simulink model "Assignment_2_PacemakerProjRA"  (R2022b)
settings: Solver=FixedStepAuto  StartTime=0.0  StopTime=30  FixedStep=1e-3  RelTol=1e-3  EnableMultiTasking=on
undefined symbols (not defined in the file): A0, A1, D0, D1, D10, D11, D12, D13, D2, D3, D4, D5, D6, D7, D8, D9, PTA0, PTA1, PTA2, PTB2, PTB23, PTB3, PTB9, PTC16, PTC17, PTC2, PTC3, PTC4, PTD0, PTD1, PTD2, PTD3
libraries: frdmk64flib x22, etargetslib x8, simulink x4
settings Model: ExtModeTrigDuration=5  Creator=varun  LastModifiedBy=lupas
settings SolverCC: AutoInsertRateTranBlk=on
settings OptimizationCC: EnhancedBackFolding=on  PassReuseOutputArgsAs=Individual arguments  ZeroExternalMemoryAtStartup=off  ZeroInternalMemoryAtStartup=off  MaxStackSize=64  OptimizeBlockOrder=speed  DifferentSizesBufferReuse=on  OptimizationCustomize=off  EfficientTunableParamExpr=on
settings DebuggingCC: ParameterTunabilityLossMsg=error
settings HardwareCC: ProdBitPerPointer=32  ProdBitPerSizeT=32  ProdBitPerPtrDiffT=32  ProdLargestAtomicInteger=Long  ProdLargestAtomicFloat=Double  ProdWordSize=32  ProdHWDeviceType=ARM Compatible->ARM Cortex
settings SFSimCC: MATLABDynamicMemAlloc=off
settings RTWCC: Description=Embedded Coder  SystemTargetFile=ert.tlc  HardwareBoard=NXP FRDM-K64F  TLCOptions="-aInlineSetEventsForThisBaseRateFcn=TLC_FALSE -aSuppressMultiTaskScheduler=TLC_FALSE  -aRateBasedStepFcn=0"  TemplateMakefile=ert_default_tmf  Toolchain=GNU Tools for ARM Embedded Processors
settings CodeAppCC: ForceParamTrailComments=on  IgnoreCustomStorageClasses=off  OperatorAnnotations=on  SimulinkDataObjDesc=on  SFDataObjDesc=on  InsertBlockDesc=on
settings ERTTargetCC: ExtModeTransport=4  ExtModeMexFile=sendToCommService

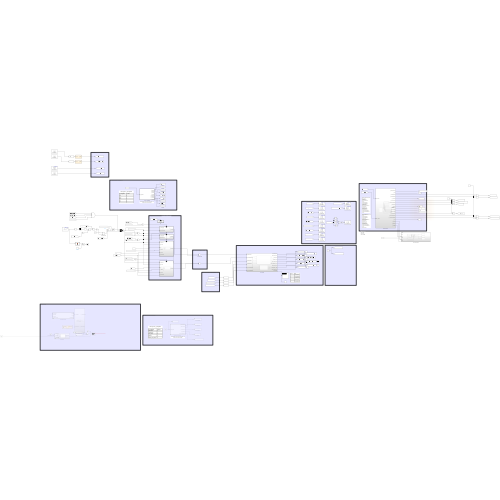
[thumbnail: Simulink's stored preview of the top-level diagram]
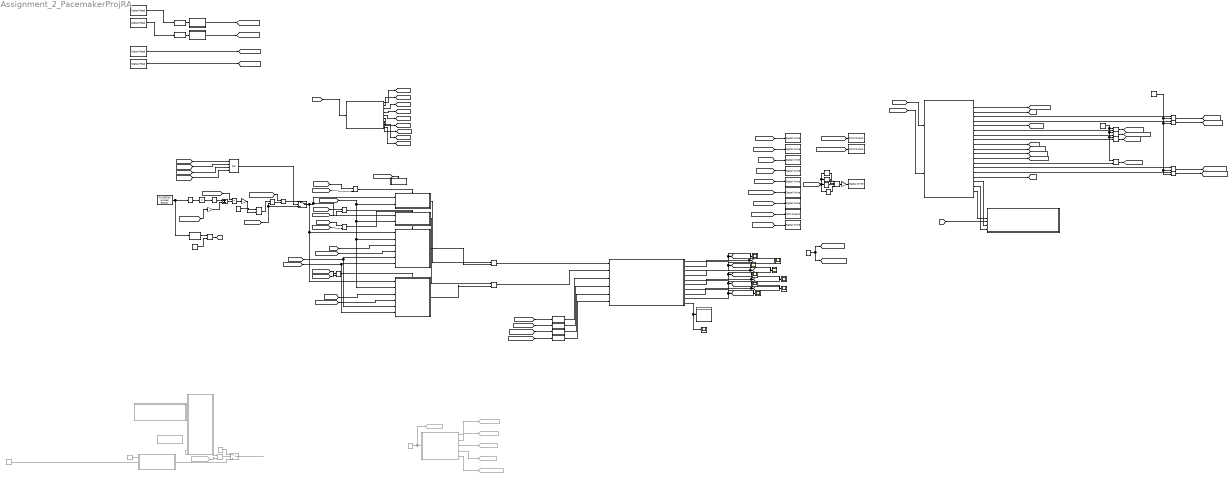
== system Assignment_2_PacemakerProjRA ==
  note: p_currentState:
      | 0x20 = Write
      | 0x16 = Echo
      | 0x22 = EGRAM
  note: Pace Making Code
  note: 'Input Variables
  note: Unused functions
  note: REF_PWM setter
  note: Output Pins
  note: Pacing System Programmable Variables
  note: Output
      | State
      |
      | 1
      | y_atriumPaced
      |
      | 2
      | y_ventriclePaced
      |
      | 3
      | y_initialDischarge
      |
      | 4
      | y_c22Charged
      |
      | 5
      | y_pulseReceived
  note: Atrial and Ventricular Pacing Signals
  note: Decoding and defining Pacing States
  note: Decoding and defining Pacing Modes
  note: Simple MATLAB code to convert input integer into a boolean set of output variables
  note: Taken from: Page 16 - Section 3.5
  note: Units/Type for y_pacingMode
      |
      | p_pacingMode
      | Int Value
      |
      | OFF
      | 0
      |
      | AOO
      | 1
      |
      | VOO
      | 2
      |
      | AAI
      | 3
      |
      | VVI
      | 4
  note: Pacing Modes
  note: Units/Type for y_pacingState
      |
      | p_pacingMode
      | Int Value
      |
      | PERMANENT
      | 0
      |
      | TEMPORARY
      | 1
      |
      | PACE_NOW
      | 2
      |
      | MAGNET
      | 3
      |
      | POWER_ON_RESET
      | 4
  note: Simple MATLAB code to convert input integer into a boolean set of output variables
  note: Number of Bytes for Input: 24
      | sync: 1 (16)
      | p_currentState: 1
      | p_mode: 1
      | p_activityThreshold: 1
      | p_arp: 2
      | p_atrialAmplitude: 2
      | p_atrialPulseWidth: 2
      | p_hysteresis: 1
      | p_hysteresisLimit: 1
      | p_maximumSensorRate: 1
      | p_lowrateLimit: 1
      | p_reactionTime: 1
      | p_recoveryTime: 1
      | p_responseFactor: 1
      | p_upperrateLimit: 1
      | p_ventricularAmplitude: 2
      | p_ventricularPulseWidth: 2
      | p_vrp: 2
  note: Input and Output for UART
  note: Number of Bytes for Output: 26
      | p_activityThreshold: 1
      | p_arp: 2
      | p_atrialAmplitude: 2
      | p_atrialPulseWidth: 2
      | p_hysteresis: 1
      | p_hysteresisLimit: 1
      | p_maximumSensorRate: 1
      | p_lowrateLimit: 1
      | p_reactionTime: 1
      | p_recoveryTime: 1
      | p_responseFactor: 1
      | p_upperrateLimit: 1
      | p_ventricularAmplitude: 2
      | p_ventricularPulseWidth: 2
      | p_vrp: 2
      | The two signals
  AAI : Subsystem
  AOO : Subsystem
  Chart : Stateflow chart  TreatAsAtomicUnit=on
  Chart1 : Stateflow chart  TreatAsAtomicUnit=on
  Compare To Constant : simulink/Logic and Bit Operations/Compare To Constant  relop===  const=3  OutDataTypeStr=boolean
  Compare To Constant1 : simulink/Logic and Bit Operations/Compare To Constant  relop===  const=4  OutDataTypeStr=boolean
  Compare To Constant2 : simulink/Logic and Bit Operations/Compare To Constant  relop===  const=7  OutDataTypeStr=boolean
  Compare To Constant3 : simulink/Logic and Bit Operations/Compare To Constant  relop===  const=8  OutDataTypeStr=boolean
  Constant : Constant  Value=0.8
  Constant1 : Constant  Value=70
  Constant19 : Constant  Commented=on  Value=0.4  OutDataTypeStr=single
  Constant20 : Constant  Commented=on  Value=.5
  Constant4 : Constant  Value=1000
  Constant5 : Constant  Value=60000
  Constant6 : Constant  Value=60000
  Cool Colour Effects : Subsystem
  Data Processing : Subsystem
  Data Type Conversion : DataTypeConversion  OutDataTypeStr=uint16  SaturateOnIntegerOverflow=off  RndMeth=Floor
  Data Type Conversion1 : DataTypeConversion  OutDataTypeStr=uint16  SaturateOnIntegerOverflow=off  RndMeth=Floor
  Data Type Conversion{2..5} (4 alike) : DataTypeConversion  OutDataTypeStr=double  SaturateOnIntegerOverflow=off  RndMeth=Floor
  Decode p_pacingMode : MATLAB Function  TreatAsAtomicUnit=on
  Decode p_pacingState : MATLAB Function  Commented=on  TreatAsAtomicUnit=on
  Digital Read : frdmk64flib/Digital Read  Whichpin=PTC16 (D0)  SampleTime=-1
  Digital Read1 : frdmk64flib/Digital Read  Whichpin=PTC17 (D1)  SampleTime=-1
  Digital Read2 : frdmk64flib/Digital Read  Whichpin=PTB2 (A0)  SampleTime=-1
  Digital Read3 : frdmk64flib/Digital Read  Whichpin=PTB3 (A1)  SampleTime=-1
  Digital Write : frdmk64flib/Digital Write  Whichpin=PTD2 (D11)
  Digital Write1 : frdmk64flib/Digital Write  Whichpin=PTD3 (D12)
  Digital Write2 : frdmk64flib/Digital Write  Whichpin=PTB23 (D4)
  Digital Write3 : frdmk64flib/Digital Write  Whichpin=PTC3 (D7)
  Digital Write4 : frdmk64flib/Digital Write  Whichpin=PTA0 (D8)
  Digital Write5 : frdmk64flib/Digital Write  Whichpin=PTB9 (D2)
  Digital Write6 : frdmk64flib/Digital Write  Whichpin=PTD0 (D10)
  Digital Write8 : frdmk64flib/Digital Write  Whichpin=PTC4 (D9)
  Digital Write9 : frdmk64flib/Digital Write  Whichpin=PTD1 (D13)
  Display : Display
  Divide{,1..7} (8 alike) : Product  Inputs=*/
  FXOS8700 6-Axes Sensor1 : frdmk64flib/FXOS8700 6-Axes Sensor  Activesensor=Accelerometer only  ODR=800Hz  HybridODR=400Hz  Accelfullrange=-4g to +4g  SampleTime=-1
  Float Variable6 : Subsystem  Commented=on
  From52 : From  Commented=on  GotoTag=s_paceNowState
  From53 : From  Commented=on  GotoTag=s_powerOnResetState
  Gain : Gain  Gain=0.5
  Gain1 : Gain  Gain=4
  Goto28 : Goto  Commented=on  GotoTag=p_currentState
  GreaterThan : RelationalOperator  OutDataTypeStr=boolean  RndMeth=Simplest  InputSameDT=off
  Lowrate Upperrate Limit Checker1 : Subsystem  Commented=on
  MATLAB Function1 : MATLAB Function  TreatAsAtomicUnit=on
  Max1 : MinMax  Inputs=2
  Min1 : MinMax  Function=max  Inputs=2
  Minus1 : Sum  Inputs=+-
  Multiply : Gain  Gain=3.3  OutDataTypeStr=double
  OFF : Subsystem
  OR : Logic  Operator=OR  Inputs=4  IconShape=distinctive  AllPortsSameDT=off  OutDataTypeStr=boolean
  OR{1..4} (4 alike) : Logic  Operator=OR  IconShape=distinctive  AllPortsSameDT=off  OutDataTypeStr=boolean
  OR5 : Logic  Operator=OR  Inputs=4  IconShape=distinctive  AllPortsSameDT=off  OutDataTypeStr=boolean
  OR8 : Logic  Commented=on  Operator=OR  IconShape=distinctive  AllPortsSameDT=off  OutDataTypeStr=boolean
  PWM Output : frdmk64flib/PWM Output  Whichpin=PTA1 (D3)  InitialFrequency=2000  InitialDutyCycle=50
  PWM Output1 : frdmk64flib/PWM Output  Whichpin=PTA2 (D5)  InitialFrequency=2000  InitialDutyCycle=50
  PWM Output2 : frdmk64flib/PWM Output  Whichpin=PTC2 (D6)  InitialFrequency=2000  InitialDutyCycle=50
  Pacing System : Subsystem
  Product : Product
  Scope{,2..10} (10 alike) : Scope
  Sqrt : Sqrt
  Square : Math  Operator=square
  Sum of Elements : Sum  Inputs=+
  Switch : Switch  Criteria=u2 > Threshold  SaturateOnIntegerOverflow=off  InputSameDT=off
  Switch7 : Switch  Commented=on  Criteria=u2 > Threshold  OutDataTypeStr=single  SaturateOnIntegerOverflow=off  InputSameDT=off
  VOO : Subsystem
  VVI : Subsystem
  Write Mode : Stateflow chart  Commented=on  TreatAsAtomicUnit=on
  checkRangeFunction7 : MATLAB Function  Commented=on  TreatAsAtomicUnit=on
  p_lowrateInterval1 : Product  Inputs=*/
  p_pacingState : Constant  Commented=on  Value=0  OutDataTypeStr=uint8
  p_ventricularPulseWidth1 : Constant  Commented=on  Value=0.4  OutDataTypeStr=single
  s_atrialPaceStart : Logic  Operator=OR  IconShape=distinctive  AllPortsSameDT=off  OutDataTypeStr=boolean
  s_magnetState : Goto  Commented=on  GotoTag=s_magnetState
  s_paceNowState : Goto  Commented=on  GotoTag=s_paceNowState
  s_permanentState : Goto  Commented=on  GotoTag=s_permanentState
  s_powerOnResetState : Goto  Commented=on  GotoTag=s_powerOnResetState
  s_temporaryState : Goto  Commented=on  GotoTag=s_temporaryState
  s_ventricularPaceStart : Logic  Operator=OR  IconShape=distinctive  AllPortsSameDT=off  OutDataTypeStr=boolean
  wires:
  [s_offState] -> OFF/Enable
  Decode p_pacingMode/1(s_offState) -> [s_offState]
  Decode p_pacingMode/2(s_AOOState) -> [s_AOOState]
  Decode p_pacingMode/4(s_AAIState) -> [s_AAIState]
  Decode p_pacingMode/5(s_VVIState) -> [s_VVIState]
  Decode p_pacingMode/3(s_VOOState) -> [s_VOOState]
  p_pacingState/1 -> Goto28/1, Decode p_pacingState/1(p_pacingState)
  Decode p_pacingState/1(s_permanentState) -> s_permanentState/1
  Decode p_pacingState/2(s_temporaryState) -> s_temporaryState/1
  Decode p_pacingState/3(s_paceNowState) -> s_paceNowState/1
  Decode p_pacingState/4(s_magnetState) -> s_magnetState/1
  Decode p_pacingState/5(S_powerOnResetState) -> s_powerOnResetState/1
  OR3/1 -> AAI/Enable
  OR4/1 -> VVI/Enable
  s_atrialPaceStart/1 -> Pacing System/1(s_atrialPaceStart)
  [p_atrialAmplitude] -> Data Type Conversion5/1
  [p_atrialPulseWidth] -> Data Type Conversion4/1
  [p_ventricularAmplitude] -> Data Type Conversion3/1
  [p_ventricularPulseWidth] -> Data Type Conversion2/1
  s_ventricularPaceStart/1 -> Pacing System/2(s_ventricularPaceStart)
  Pacing System/1(ATR_GND_CTRL) -> [ATR_GND_CTRL], Scope2/1
  Pacing System/3(Z_ATR_CTRL) -> [Z_ATR_CTRL], Scope4/1
  Pacing System/2(VENT_GND_CTRL) -> [VENT_GND_CTRL], Scope3/1
  Pacing System/4(Z_VENT_CTRL) -> Scope5/1, [Z_VENT_CTRL]
  Pacing System/6(PACE_CHARGE_CTRL) -> Scope7/1, [PACE_CHARGE_CTRL]
  Pacing System/5(ATR_PACE_CTRL) -> [ATR_PACE_CTRL], Scope6/1
  Pacing System/7(PACE_GND_CTRL) -> Scope8/1, [PACE_GND_CTRL]
  Pacing System/9(VENT_PACE_CTRL) -> [VENT_PACE_CTRL], Scope10/1
  Pacing System/8(PACING_REF_PWM) -> Scope9/1, [PACING_REF_PWM]
  Pacing System/10(Visual Output) -> Scope/1, Display/1
  [VENT_PACE_CTRL] -> Digital Write8/1
  [PACING_REF_PWM] -> PWM Output1/1
  [PACE_GND_CTRL] -> Digital Write6/1
  [PACE_CHARGE_CTRL] -> Digital Write5/1
  [ATR_PACE_CTRL] -> Digital Write4/1
  [Z_VENT_CTRL] -> Digital Write3/1
  [Z_ATR_CTRL] -> Digital Write2/1
  [VENT_GND_CTRL] -> Digital Write1/1
  [ATR_GND_CTRL] -> Digital Write/1
  OR1/1 -> AOO/Enable
  OR2/1 -> VOO/Enable
  AOO/1(s_paceStart) -> s_atrialPaceStart/1
  VOO/1(s_paceStart) -> s_ventricularPaceStart/1
  Digital Read/1 -> [ATR_CMP_DETECT]
  Digital Read1/1 -> [VENT_CMP_DETECT]
  [ATR_CMP_REF_PWM] -> PWM Output2/1
  [VENT_CMP_REF_PWM] -> PWM Output/1
  Constant1/1 -> [ATR_CMP_REF_PWM], [VENT_CMP_REF_PWM]
  OR/1 -> Multiply/1
  Compare To Constant/1 -> OR/1
  Compare To Constant1/1 -> OR/2
  Multiply/1 -> Digital Write9/1
  [p_mode] -> Compare To Constant3/1, Compare To Constant2/1, Compare To Constant1/1, Compare To Constant/1
  AAI/1(s_paceStart) -> s_atrialPaceStart/2
  VVI/1(s_paceStart) -> s_ventricularPaceStart/2
  [p_upperrateLimit] -> AOO/2(p_uppperrateInterval), VOO/2(p_uppperrateInterval), VVI/2(p_upperLimit), AAI/2(p_upperLimit)
  [ATR_CMP_DETECT] -> AAI/4(m_atrSense)
  [p_arp] -> AAI/3(p_arp)
  [p_vrp] -> VVI/3(p_vrp)
  [VENT_CMP_DETECT] -> VVI/4(m_ventSense)
  Data Type Conversion2/1 -> Pacing System/6(p_ventricularPulseWidth)
  Data Type Conversion3/1 -> Pacing System/5(p_ventricularAmplitude)
  Data Type Conversion4/1 -> Pacing System/4(p_atrialPulseWidth)
  Data Type Conversion5/1 -> Pacing System/3(p_atrialAmplitude)
  Constant20/1 -> Switch7/1
  Float Variable6/1(p_outputValue) -> Switch7/3
  From53/1 -> OR8/1
  OR8/1 -> Switch7/2
  From52/1 -> OR8/2
  Constant19/1 -> Float Variable6/2(m_newValue)
  p_ventricularPulseWidth1/1 -> Float Variable6/1(k_defaultValue)
  Switch7/1 -> ?
  [p_mode] -> Decode p_pacingMode/1(p_pacingMode)
  Divide2/1 -> [p_upperrateLimit]
  Divide1/1 -> [p_maximumSensorRate]
  Divide/1 -> [p_lowrateLimit]
  Constant5/1 -> Divide7/1, Divide2/1, Divide/1, Divide1/1
  Data Processing/1(p_activityThreshold1) -> [p_activityThreshold]
  Data Processing/2(p_arp1) -> [p_arp]
  Data Processing/3(p_atrialAmplitude1) -> Divide3/1
  Data Processing/4(p_atrialPulseWidth1) -> Divide4/1
  Data Processing/5(p_hysteresis1) -> [p_hysteresis]
  Data Processing/7(p_maximumSensorRate1) -> Divide1/2
  Data Processing/8(p_lowrateLimit1) -> Divide/2
  Data Processing/10(p_reactionTime1) -> [p_reactionTime]
  Data Processing/11(p_recoveryTime1) -> [p_recoveryTime]
  Data Processing/12(p_responseFactor1) -> [p_responseFactor]
  Data Processing/13(p_upperrateLimit1) -> Divide2/2
  Data Processing/14(p_ventricularAmplitude1) -> Divide5/1
  Data Processing/15(p_ventricularPulseWidth1) -> Divide6/1
  Data Processing/16(p_vrp1) -> [p_vrp]
  Data Processing/18(p_uartGreen) -> Cool Colour Effects/6(Green)
  Data Processing/19(p_uartBlue) -> Cool Colour Effects/3(Blue)
  Data Processing/17(p_uartRed) -> Cool Colour Effects/5(Red)
  Data Processing/9(p_mode1) -> [p_mode]
  Divide3/1 -> [p_atrialAmplitude]
  Divide4/1 -> [p_atrialPulseWidth]
  Constant4/1 -> Divide6/2, Divide5/2, Divide4/2, Divide3/2
  Divide6/1 -> [p_ventricularPulseWidth]
  Divide5/1 -> [p_ventricularAmplitude]
  Data Processing/6(p_hysteresisLimit1) -> Divide7/2
  [p_hysteresis] -> VVI/5(p_hysteresis), AAI/5(p_hysteresis)
  [p_hysteresisLimit] -> VVI/6(p_hysteresisLimit), AAI/6(p_hysteresisLimit)
  Digital Read3/1 -> Data Type Conversion1/1
  Digital Read2/1 -> Data Type Conversion/1
  [ATR_SIGNAL] -> Data Processing/1(ATR_SIGNAL)
  [VENT_SIGNAL] -> Data Processing/2(VENT_SIGNAL)
  Divide7/1 -> [p_hysteresisLimit]
  Data Type Conversion/1 -> Chart/1(m_input)
  Data Type Conversion1/1 -> Chart1/1(m_input)
  Chart/1(p_output) -> [ATR_SIGNAL]
  Chart1/1(p_output) -> [VENT_SIGNAL]
  Decode p_pacingMode/6(s_AOORState) -> [s_AOORState]
  Decode p_pacingMode/7(s_VOORState) -> [s_VOORState]
  Decode p_pacingMode/8(s_AAIRState) -> [s_AAIRState]
  Decode p_pacingMode/9(s_VVIRState) -> [s_VVIRState]
  [s_AOOState] -> OR1/2
  [s_AOORState] -> OR1/1
  [s_VOOState] -> OR2/2
  [s_VOORState] -> OR2/1
  [s_AAIState] -> OR3/2
  [s_AAIRState] -> OR3/1
  [s_VVIState] -> OR4/1
  [s_VVIRState] -> OR4/2
  [s_VVIRState] -> OR5/4
  [s_AAIRState] -> OR5/3
  [s_VOORState] -> OR5/2
  [s_AOORState] -> OR5/1
  Compare To Constant2/1 -> OR/3
  Compare To Constant3/1 -> OR/4
  FXOS8700 6-Axes Sensor1/1 -> MATLAB Function1/1(u), Square/1
  MATLAB Function1/1(y) -> GreaterThan/1
  GreaterThan/1 -> [SUS]
  Constant/1 -> GreaterThan/2
  [SUS] -> Cool Colour Effects/4(Yellow)
  OR5/1 -> Switch/2
  Minus1/1 -> Product/2
  [p_maximumSensorRate] -> Min1/1
  Constant6/1 -> p_lowrateInterval1/1
  Product/1 -> Gain1/1
  Sqrt/1 -> Minus1/1
  Square/1 -> Sum of Elements/1
  Max1/1 -> Min1/2
  [p_lowrateLimit] -> Switch/3, Max1/2
  Sum of Elements/1 -> Sqrt/1
  [p_responseFactor] -> Product/1
  Gain/1 -> Minus1/2
  [p_activityThreshold] -> Gain/1
  Gain1/1 -> p_lowrateInterval1/2
  p_lowrateInterval1/1 -> Max1/1
  Min1/1 -> Switch/1
  Switch/1 -> VVI/1(p_lowrateLimit), AAI/1(p_lowrateLimit), VOO/1(p_lowrateInterval), AOO/1(p_lowrateInterval)

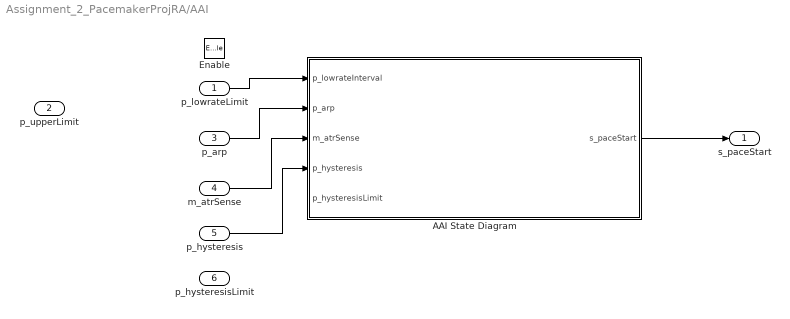
== system Assignment_2_PacemakerProjRA/AAI ==
  p_lowrateLimit : Inport
  p_upperLimit : Inport  Port=2
  p_arp : Inport  Port=3
  m_atrSense : Inport  Port=4
  p_hysteresis : Inport  Port=5
  p_hysteresisLimit : Inport  Port=6
  Enable : EnablePort
  AAI State Diagram : Stateflow chart  TreatAsAtomicUnit=on
  s_paceStart : Outport
  wires:
  p_lowrateLimit/1 -> AAI State Diagram/1(p_lowrateInterval)
  AAI State Diagram/1(s_paceStart) -> s_paceStart/1
  m_atrSense/1 -> AAI State Diagram/3(m_atrSense)
  p_arp/1 -> AAI State Diagram/2(p_arp)
  p_hysteresis/1 -> AAI State Diagram/4(p_hysteresis)

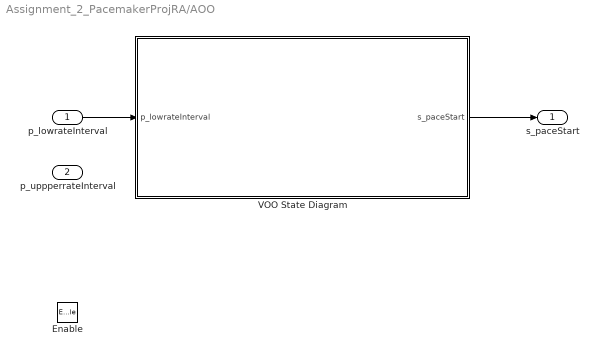
== system Assignment_2_PacemakerProjRA/AOO ==
  p_lowrateInterval : Inport
  p_uppperrateInterval : Inport  Port=2
  Enable : EnablePort
  VOO State Diagram : Stateflow chart  TreatAsAtomicUnit=on
  s_paceStart : Outport
  wires:
  p_lowrateInterval/1 -> VOO State Diagram/1(p_lowrateInterval)
  VOO State Diagram/1(s_paceStart) -> s_paceStart/1

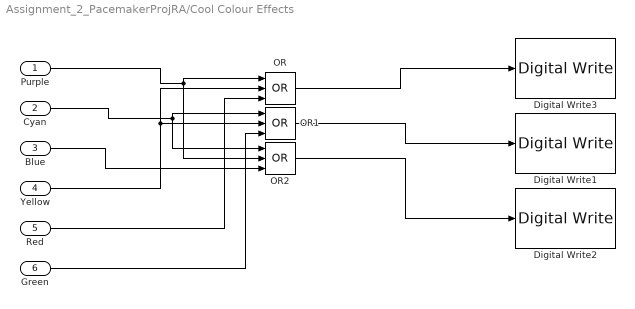
== system Assignment_2_PacemakerProjRA/Cool Colour Effects ==
  Purple : Inport
  Cyan : Inport  Port=2
  Blue : Inport  Port=3
  Yellow : Inport  Port=4
  Red : Inport  Port=5
  Green : Inport  Port=6
  Digital Write1 : frdmk64flib/Digital Write  Whichpin=GREEN_LED
  Digital Write2 : frdmk64flib/Digital Write  Whichpin=BLUE_LED
  Digital Write3 : frdmk64flib/Digital Write  Whichpin=RED_LED
  OR : Logic  Operator=OR  Inputs=3  IconShape=distinctive  AllPortsSameDT=off  OutDataTypeStr=boolean
  OR1 : Logic  Operator=OR  Inputs=3  IconShape=distinctive  AllPortsSameDT=off  OutDataTypeStr=boolean
  OR2 : Logic  Operator=OR  Inputs=3  IconShape=distinctive  AllPortsSameDT=off  OutDataTypeStr=boolean
  wires:
  Blue/1 -> OR2/3
  Cyan/1 -> OR2/1, OR1/1
  Purple/1 -> OR2/2, OR/1
  Yellow/1 -> OR1/2, OR/2
  Red/1 -> OR/3
  Green/1 -> OR1/3
  OR/1 -> Digital Write3/1
  OR2/1 -> Digital Write2/1
  OR1/1 -> Digital Write1/1

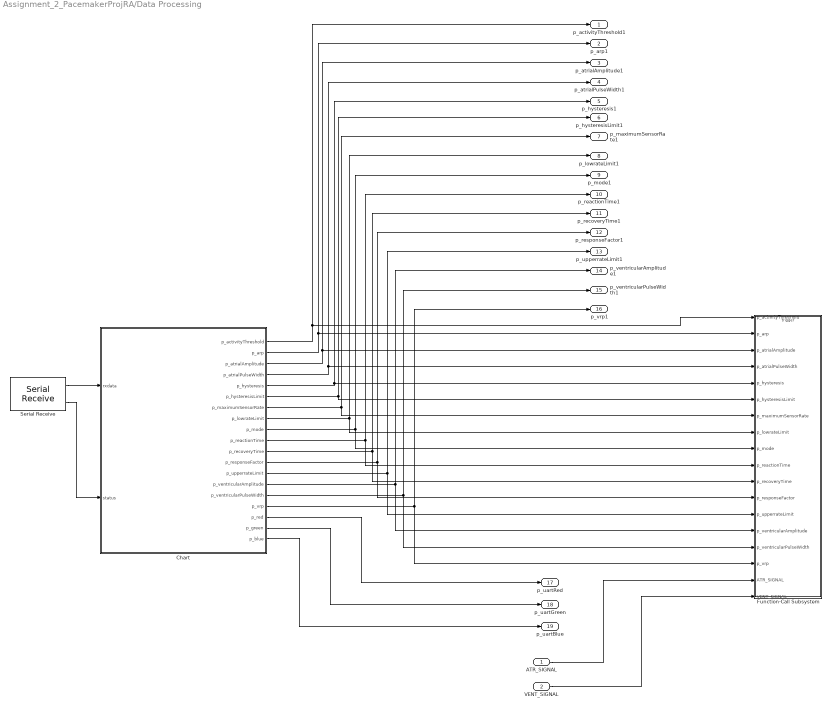
== system Assignment_2_PacemakerProjRA/Data Processing ==
  ATR_SIGNAL : Inport  OutDataTypeStr=uint16
  VENT_SIGNAL : Inport  Port=2  OutDataTypeStr=uint16
  Chart : Stateflow chart  TreatAsAtomicUnit=on
  Function-Call Subsystem : Subsystem  TreatAsAtomicUnit=on
  Serial Receive : frdmk64flib/Serial Receive  SCIModule=0  Baudrate=uint32(9600)  Parity=None  StopBits=1  HardwareFlowControl=None  ByteOrder=LittleEndian  DataType=uint8  DataLength=24  BlockingMode=off  OutputStatus=on  SampleTime=0.1
  p_activityThreshold1 : Outport
  p_arp1 : Outport  Port=2
  p_atrialAmplitude1 : Outport  Port=3
  p_atrialPulseWidth1 : Outport  Port=4
  p_hysteresis1 : Outport  Port=5
  p_hysteresisLimit1 : Outport  Port=6
  p_maximumSensorRate1 : Outport  Port=7
  p_lowrateLimit1 : Outport  Port=8
  p_mode1 : Outport  Port=9
  p_reactionTime1 : Outport  Port=10
  p_recoveryTime1 : Outport  Port=11
  p_responseFactor1 : Outport  Port=12
  p_upperrateLimit1 : Outport  Port=13
  p_ventricularAmplitude1 : Outport  Port=14
  p_ventricularPulseWidth1 : Outport  Port=15
  p_vrp1 : Outport  Port=16
  p_uartRed : Outport  Port=17
  p_uartGreen : Outport  Port=18
  p_uartBlue : Outport  Port=19
  wires:
  Serial Receive/1 -> Chart/1(rxdata)
  Serial Receive/2 -> Chart/2(status)
  Chart/17(p_red) -> p_uartRed/1
  Chart/18(p_green) -> p_uartGreen/1
  Chart/19(p_blue) -> p_uartBlue/1
  Chart/11(p_recoveryTime) -> p_recoveryTime1/1, Function-Call Subsystem/11(p_recoveryTime)
  Chart/14(p_ventricularAmplitude) -> p_ventricularAmplitude1/1, Function-Call Subsystem/14(p_ventricularAmplitude)
  Chart/3(p_atrialAmplitude) -> p_atrialAmplitude1/1, Function-Call Subsystem/3(p_atrialAmplitude)
  Chart/2(p_arp) -> p_arp1/1, Function-Call Subsystem/2(p_arp)
  Chart/7(p_maximumSensorRate) -> p_maximumSensorRate1/1, Function-Call Subsystem/7(p_maximumSensorRate)
  Chart/15(p_ventricularPulseWidth) -> p_ventricularPulseWidth1/1, Function-Call Subsystem/15(p_ventricularPulseWidth)
  Chart/9(p_mode) -> p_mode1/1, Function-Call Subsystem/9(p_mode)
  Chart/8(p_lowrateLimit) -> p_lowrateLimit1/1, Function-Call Subsystem/8(p_lowrateLimit)
  Chart/4(p_atrialPulseWidth) -> p_atrialPulseWidth1/1, Function-Call Subsystem/4(p_atrialPulseWidth)
  Chart/13(p_upperrateLimit) -> p_upperrateLimit1/1, Function-Call Subsystem/13(p_upperrateLimit)
  Chart/12(p_responseFactor) -> p_responseFactor1/1, Function-Call Subsystem/12(p_responseFactor)
  Chart/1(p_activityThreshold) -> p_activityThreshold1/1, Function-Call Subsystem/1(p_activityThreshold)
  Chart/5(p_hysteresis) -> p_hysteresis1/1, Function-Call Subsystem/5(p_hysteresis)
  Chart/16(p_vrp) -> p_vrp1/1, Function-Call Subsystem/16(p_vrp)
  Chart/10(p_reactionTime) -> p_reactionTime1/1, Function-Call Subsystem/10(p_reactionTime)
  Chart/6(p_hysteresisLimit) -> p_hysteresisLimit1/1, Function-Call Subsystem/6(p_hysteresisLimit)
  ATR_SIGNAL/1 -> Function-Call Subsystem/17(ATR_SIGNAL)
  VENT_SIGNAL/1 -> Function-Call Subsystem/18(VENT_SIGNAL)

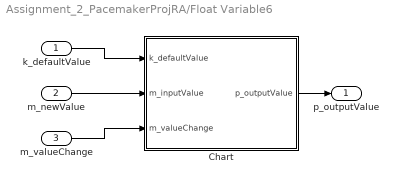
== system Assignment_2_PacemakerProjRA/Float Variable6 ==
  k_defaultValue : Inport
  m_newValue : Inport  Port=2
  m_valueChange : Inport  Port=3
  Chart : Stateflow chart  TreatAsAtomicUnit=on
  p_outputValue : Outport
  wires:
  Chart/1(p_outputValue) -> p_outputValue/1
  m_newValue/1 -> Chart/2(m_inputValue)
  k_defaultValue/1 -> Chart/1(k_defaultValue)
  m_valueChange/1 -> Chart/3(m_valueChange)

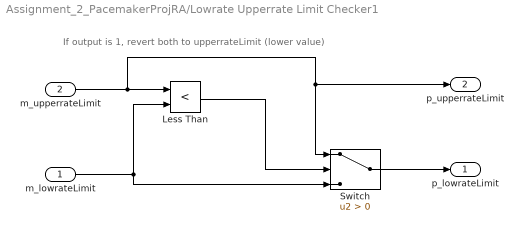
== system Assignment_2_PacemakerProjRA/Lowrate Upperrate Limit Checker1 ==
  note: If output is 1, revert both to upperrateLimit (lower value)
  m_lowrateLimit : Inport
  m_upperrateLimit : Inport  Port=2
  Less Than : RelationalOperator  Operator=<  OutDataTypeStr=boolean  RndMeth=Simplest  InputSameDT=off
  Switch : Switch  Criteria=u2 > Threshold  SaturateOnIntegerOverflow=off  InputSameDT=off
  p_lowrateLimit : Outport  OutDataTypeStr=single
  p_upperrateLimit : Outport  Port=2  OutDataTypeStr=single
  wires:
  m_upperrateLimit/1 -> Switch/1, p_upperrateLimit/1, Less Than/1
  m_lowrateLimit/1 -> Switch/3, Less Than/2
  Switch/1 -> p_lowrateLimit/1
  Less Than/1 -> Switch/2

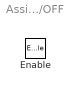
== system Assignment_2_PacemakerProjRA/OFF ==
  Enable : EnablePort

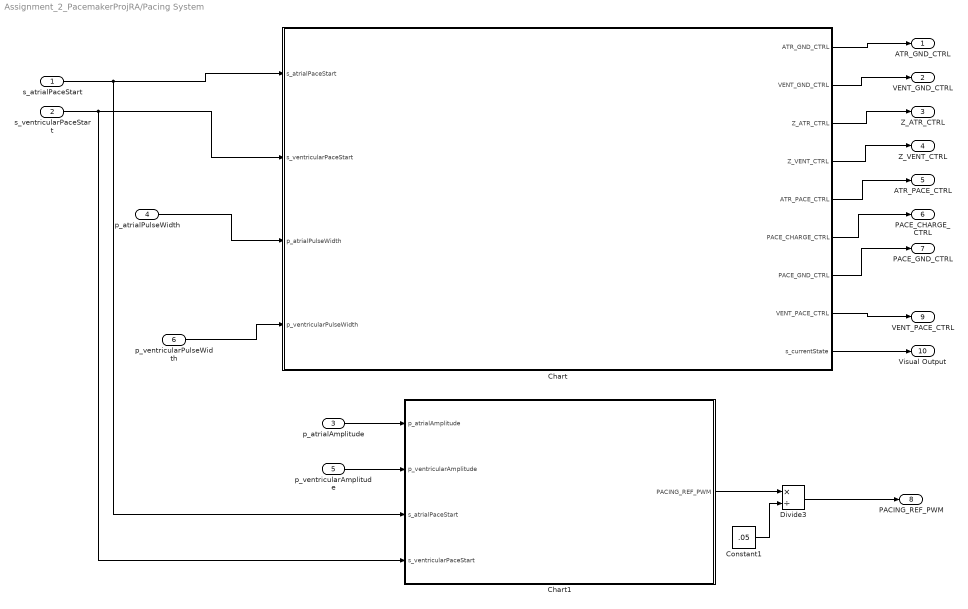
== system Assignment_2_PacemakerProjRA/Pacing System ==
  s_atrialPaceStart : Inport
  s_ventricularPaceStart : Inport  Port=2
  p_atrialAmplitude : Inport  Port=3
  p_atrialPulseWidth : Inport  Port=4
  p_ventricularAmplitude : Inport  Port=5  OutDataTypeStr=double
  p_ventricularPulseWidth : Inport  Port=6  OutDataTypeStr=double
  Chart : Stateflow chart  TreatAsAtomicUnit=on
  Chart1 : Stateflow chart  TreatAsAtomicUnit=on
  Constant1 : Constant  Value=.05  OutDataTypeStr=double
  Divide3 : Product  Inputs=*/
  ATR_GND_CTRL : Outport
  VENT_GND_CTRL : Outport  Port=2
  Z_ATR_CTRL : Outport  Port=3
  Z_VENT_CTRL : Outport  Port=4
  ATR_PACE_CTRL : Outport  Port=5
  PACE_CHARGE_CTRL : Outport  Port=6
  PACE_GND_CTRL : Outport  Port=7
  PACING_REF_PWM : Outport  Port=8
  VENT_PACE_CTRL : Outport  Port=9
  Visual Output : Outport  Port=10
  wires:
  s_atrialPaceStart/1 -> Chart1/3(s_atrialPaceStart), Chart/1(s_atrialPaceStart)
  s_ventricularPaceStart/1 -> Chart1/4(s_ventricularPaceStart), Chart/2(s_ventricularPaceStart)
  p_atrialPulseWidth/1 -> Chart/3(p_atrialPulseWidth)
  Chart/1(ATR_GND_CTRL) -> ATR_GND_CTRL/1
  Chart/2(VENT_GND_CTRL) -> VENT_GND_CTRL/1
  Chart/3(Z_ATR_CTRL) -> Z_ATR_CTRL/1
  Chart/4(Z_VENT_CTRL) -> Z_VENT_CTRL/1
  Chart/5(ATR_PACE_CTRL) -> ATR_PACE_CTRL/1
  Chart/6(PACE_CHARGE_CTRL) -> PACE_CHARGE_CTRL/1
  Chart/7(PACE_GND_CTRL) -> PACE_GND_CTRL/1
  Chart/8(VENT_PACE_CTRL) -> VENT_PACE_CTRL/1
  Chart/9(s_currentState) -> Visual Output/1
  p_ventricularPulseWidth/1 -> Chart/4(p_ventricularPulseWidth)
  p_ventricularAmplitude/1 -> Chart1/2(p_ventricularAmplitude)
  p_atrialAmplitude/1 -> Chart1/1(p_atrialAmplitude)
  Chart1/1(PACING_REF_PWM) -> Divide3/1
  Constant1/1 -> Divide3/2
  Divide3/1 -> PACING_REF_PWM/1

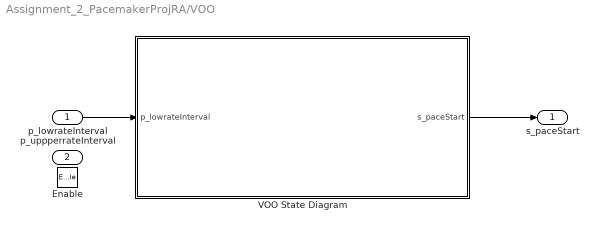
== system Assignment_2_PacemakerProjRA/VOO ==
  p_lowrateInterval : Inport
  p_uppperrateInterval : Inport  Port=2
  Enable : EnablePort
  VOO State Diagram : Stateflow chart  TreatAsAtomicUnit=on
  s_paceStart : Outport
  wires:
  p_lowrateInterval/1 -> VOO State Diagram/1(p_lowrateInterval)
  VOO State Diagram/1(s_paceStart) -> s_paceStart/1

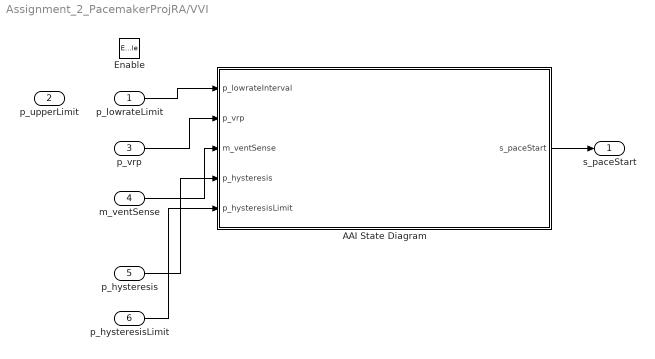
== system Assignment_2_PacemakerProjRA/VVI ==
  p_lowrateLimit : Inport
  p_upperLimit : Inport  Port=2
  p_vrp : Inport  Port=3
  m_ventSense : Inport  Port=4
  p_hysteresis : Inport  Port=5
  p_hysteresisLimit : Inport  Port=6
  Enable : EnablePort
  AAI State Diagram : Stateflow chart  TreatAsAtomicUnit=on
  s_paceStart : Outport
  wires:
  AAI State Diagram/1(s_paceStart) -> s_paceStart/1
  p_lowrateLimit/1 -> AAI State Diagram/1(p_lowrateInterval)
  p_vrp/1 -> AAI State Diagram/2(p_vrp)
  m_ventSense/1 -> AAI State Diagram/3(m_ventSense)
  p_hysteresis/1 -> AAI State Diagram/4(p_hysteresis)
  p_hysteresisLimit/1 -> AAI State Diagram/5(p_hysteresisLimit)

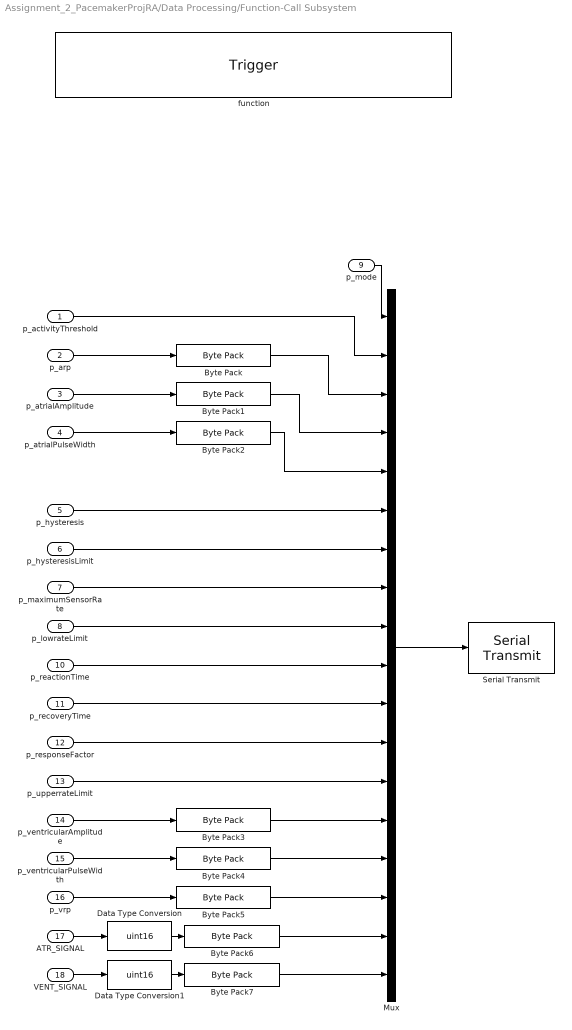
== system Assignment_2_PacemakerProjRA/Data Processing/Function-Call Subsystem ==
  p_activityThreshold : Inport
  p_arp : Inport  Port=2
  p_atrialAmplitude : Inport  Port=3
  p_atrialPulseWidth : Inport  Port=4
  p_hysteresis : Inport  Port=5
  p_hysteresisLimit : Inport  Port=6
  p_maximumSensorRate : Inport  Port=7
  p_lowrateLimit : Inport  Port=8
  p_mode : Inport  Port=9
  p_reactionTime : Inport  Port=10
  p_recoveryTime : Inport  Port=11
  p_responseFactor : Inport  Port=12
  p_upperrateLimit : Inport  Port=13
  p_ventricularAmplitude : Inport  Port=14
  p_ventricularPulseWidth : Inport  Port=15
  p_vrp : Inport  Port=16
  ATR_SIGNAL : Inport  Port=17
  VENT_SIGNAL : Inport  Port=18
  function : TriggerPort  TriggerType=function-call  IsSimulinkFunction=on  FunctionName=echo_params_alt  VariantControl=(inherit)
  Byte Pack{,1..7} (8 alike) : etargetslib/Byte Pack  datatypes={'uint16'}  byteAlign=1
  Data Type Conversion : DataTypeConversion  OutDataTypeStr=uint16  SaturateOnIntegerOverflow=off  RndMeth=Floor
  Data Type Conversion1 : DataTypeConversion  OutDataTypeStr=uint16  SaturateOnIntegerOverflow=off  RndMeth=Floor
  Mux : Mux  Inputs=18
  Serial Transmit : frdmk64flib/Serial Transmit  SCIModule=0  Baudrate=uint32(9600)  Parity=None  StopBits=1  HardwareFlowControl=None  ByteOrder=LittleEndian  BlockingMode=on  OutputStatus=off
  wires:
  p_recoveryTime/1 -> Mux/11
  p_ventricularPulseWidth/1 -> Byte Pack4/1
  p_reactionTime/1 -> Mux/10
  Byte Pack/1 -> Mux/3
  Byte Pack4/1 -> Mux/15
  p_arp/1 -> Byte Pack/1
  Byte Pack5/1 -> Mux/16
  p_responseFactor/1 -> Mux/12
  Byte Pack2/1 -> Mux/5
  Byte Pack1/1 -> Mux/4
  p_atrialAmplitude/1 -> Byte Pack1/1
  p_mode/1 -> Mux/1
  p_upperrateLimit/1 -> Mux/13
  p_activityThreshold/1 -> Mux/2
  p_ventricularAmplitude/1 -> Byte Pack3/1
  p_maximumSensorRate/1 -> Mux/8
  Byte Pack3/1 -> Mux/14
  p_hysteresis/1 -> Mux/6
  p_lowrateLimit/1 -> Mux/9
  Mux/1 -> Serial Transmit/1
  p_atrialPulseWidth/1 -> Byte Pack2/1
  p_vrp/1 -> Byte Pack5/1
  p_hysteresisLimit/1 -> Mux/7
  ATR_SIGNAL/1 -> Data Type Conversion/1
  VENT_SIGNAL/1 -> Data Type Conversion1/1
  Data Type Conversion/1 -> Byte Pack6/1
  Data Type Conversion1/1 -> Byte Pack7/1
  Byte Pack6/1 -> Mux/17
  Byte Pack7/1 -> Mux/18

== matlab function Assignment_2_PacemakerProjRA/Decode p_pacingState ==
  data: p_pacingState input; s_permanentState output; s_temporaryState output; s_paceNowState output; s_magnetState output; S_powerOnResetState output
function [s_permanentState,s_temporaryState, s_paceNowState, s_magnetState, S_powerOnResetState] = decodeInputInteger(p_pacingState)

stateList = zeros(1,5);

stateList(p_pacingState + 1) = 1;

s_permanentState = stateList(1);
s_temporaryState = stateList(2);
s_paceNowState = stateList(3);
s_magnetState = stateList(4);
S_powerOnResetState = stateList(5);

== stateflow chart Assignment_2_PacemakerProjRA/Pacing System/Chart ==
  note: Step 1
  state chargingPrimaryCapacitor
    entry:
    % As per Section 3.3.1
    % To ensure atr/vent are discharged
    % upon initial start
    ATR_PACE_CTRL = false;
    VENT_PACE_CTRL = false;
    PACE_CHARGE_CTRL = true;
    PACE_GND_CTRL=true;
  state initalState
    entry:
    % x_GND_CTRL is disabled
    ATR_GND_CTRL = false;
    VENT_GND_CTRL = false;
    % Z_x_CTRL is also disabled
    Z_ATR_CTRL = false;
    Z_VENT_CTRL = false;
  state chargingBuffer
    exit:
    s_currentState = 4; % y_c22Charged
  state pacingBuffer
    exit:
    s_currentState = 5; % y_pulseReceived
  note: Step 2
  state atrialPacing
    entry:
    % As per Section 3.3.2
    PACE_CHARGE_CTRL = false;
    % PACE_GND_CTRL = true;
    ATR_PACE_CTRL = true;
    ATR_GND_CTRL = false;
    Z_ATR_CTRL = false;
    Z_VENT_CTRL = false;
    VENT_GND_CTRL = false;
    VENT_PACE_CTRL = false;
    exit:
    s_currentState = 1; % y_atriumPaced
  state ventricularPacing
    entry:
    % As per Section 3.3.2
    PACE_CHARGE_CTRL = false;
    % PACE_GND_CTRL = true;
    ATR_PACE_CTRL = false;
    ATR_GND_CTRL = false;
    Z_ATR_CTRL = false;
    Z_VENT_CTRL = false;
    VENT_GND_CTRL = false;
    VENT_PACE_CTRL = true;
    exit:
    s_currentState = 2; % y_ventriclePaced
  state dischargingAtrialBlockCapacitor
    entry:
    % Do steps common to Step 3 and Step 1 here
    % PACE_GND_CTRL = true;
    % VENT_PACE_CTRL = false;
    % Z_ATR_CTRL = false;
    % Z_VENT_CTRL = false;
    ATR_PACE_CTRL = false;
    % Step unique to ventricular pacing
    % VENT_GND_CTRL = false;
    ATR_GND_CTRL = true;
    exit:
    s_currentState = 3; % y_initialDischarge
  note: Step 3
  state dischargingVentricularBlockCapacitor
    entry:
    % Do steps common to Step 3 and Step 1 here
    % PACE_GND_CTRL = true;
    VENT_PACE_CTRL = false;
    % Z_ATR_CTRL = false;
    % Z_VENT_CTRL = false;
    % ATR_PACE_CTRL = false;
    % ATR_GND_CTRL = false;
    % Step unique to ventricular pacing
    % ATR_GND_CTRL = false;
    VENT_GND_CTRL = true;
    exit:
    s_currentState = 3; % y_initialDischarge
  pacingBuffer -> ventricularPacing [order 2] : [s_atrialPaceStart == false && s_ventricularPaceStart == true]
  (default) -> initalState
  initalState -> chargingPrimaryCapacitor
  pacingBuffer -> atrialPacing [order 1] : [s_atrialPaceStart == true && s_ventricularPaceStart == false]
  chargingPrimaryCapacitor -> chargingBuffer : [s_atrialPaceStart == false && s_ventricularPaceStart == false]
  chargingBuffer -> pacingBuffer
  dischargingVentricularBlockCapacitor -> chargingPrimaryCapacitor
  dischargingAtrialBlockCapacitor -> chargingPrimaryCapacitor
  atrialPacing -> dischargingAtrialBlockCapacitor : after(p_atrialPulseWidth,msec)
  ventricularPacing -> dischargingVentricularBlockCapacitor : after(p_ventricularPulseWidth,msec)
  data: ATR_GND_CTRL output; VENT_GND_CTRL output; Z_ATR_CTRL output; Z_VENT_CTRL output; ATR_PACE_CTRL output; PACE_CHARGE_CTRL output; PACE_GND_CTRL output; VENT_PACE_CTRL output; s_atrialPaceStart input; s_ventricularPaceStart input; p_atrialPulseWidth input; p_ventricularPulseWidth input; s_currentState output

== stateflow chart Assignment_2_PacemakerProjRA/Pacing System/Chart1 ==
  state initialState
    entry:
    PACING_REF_PWM = 0;
  state atrialPacing
    entry:
    PACING_REF_PWM = p_atrialAmplitude;
  state ventricularPacing
    entry:
    PACING_REF_PWM = p_ventricularAmplitude;
  (default) -> initialState
  initialState -> atrialPacing [order 1] : [s_atrialPaceStart == true && s_ventricularPaceStart == false]
  initialState -> ventricularPacing [order 2] : [s_atrialPaceStart == false && s_ventricularPaceStart == true]
  atrialPacing -> ventricularPacing : [s_atrialPaceStart == false && s_ventricularPaceStart == true]
  ventricularPacing -> atrialPacing : [s_atrialPaceStart == true && s_ventricularPaceStart == false]
  data: PACING_REF_PWM output; p_atrialAmplitude input; p_ventricularAmplitude input; s_atrialPaceStart input; s_ventricularPaceStart input

== stateflow chart Assignment_2_PacemakerProjRA/Chart ==
  state SIGNAL
    entry:
    p_output = m_input
  state INITIAL
    entry:
    p_output = 0;
  (default) -> INITIAL
  INITIAL -> SIGNAL : [m_input > 0.5]
  SIGNAL -> INITIAL : after(100, msec)
  data: m_input input uint16; p_output output uint16

== stateflow chart Assignment_2_PacemakerProjRA/VOO/VOO State Diagram ==
  state NO_PACE
    entry:
    s_paceStart = true;
  state PACE
    entry:
    s_paceStart = false;
  (default) -> NO_PACE
  PACE -> NO_PACE : after(p_lowrateInterval, msec)
  NO_PACE -> PACE : after(1, msec)
  data: p_lowrateInterval input; s_paceStart output

== stateflow chart Assignment_2_PacemakerProjRA/AAI/AAI State Diagram ==
  state INITIAL_STATE
  state SENSED
  note: Hysteresis
  state HYSTERESIS_STATE
  state PACED
    entry:
    s_paceStart = 1;
    on after(1, msec):
    s_paceStart = 0;
  state REGULAR_STATE
  note: No Hysteresis
  (junction 47) -> SENSED
  REGULAR_STATE -> (junction 47) [order 1] : [m_atrSense]
  HYSTERESIS_STATE -> (junction 47) [order 1] : [m_atrSense]
  (default) -> INITIAL_STATE
  INITIAL_STATE -> PACED
  SENSED -> (junction 59) : after(p_arp, msec)
  (junction 59) -> HYSTERESIS_STATE [order 1] : [p_hysteresis == 1]
  HYSTERESIS_STATE -> (junction 53) [order 2] : after(p_hysteresisLimit, msec)
  REGULAR_STATE -> (junction 53) [order 2] : after(p_lowrateInterval - p_arp, msec)
  (junction 53) -> PACED
  (junction 59) -> REGULAR_STATE [order 2]
  PACED -> REGULAR_STATE : after(p_arp, msec)
  data: p_lowrateInterval input; p_arp input; s_paceStart output; m_atrSense input; p_hysteresis input; p_hysteresisLimit input

== stateflow chart Assignment_2_PacemakerProjRA/Chart1 ==
  state SIGNAL
    entry:
    p_output = m_input
  state INITIAL
    entry:
    p_output = 0;
  (default) -> INITIAL
  INITIAL -> SIGNAL : [m_input > 0.5]
  SIGNAL -> INITIAL : after(100, msec)
  data: m_input input uint16; p_output output uint16

== matlab function Assignment_2_PacemakerProjRA/checkRangeFunction7 ==
  data: m_inputValue input; p_output output; k_maxValue input; k_minValue input; k_valueNameString input; p_error output; p_errorMessage output
function [p_output, p_error, p_errorMessage] = checkRange(m_inputValue, k_maxValue, k_minValue, k_valueNameString)

if (m_inputValue > k_maxValue)
    p_error = 1;
    p_errorMessage = k_valueNameString;
    p_output = k_maxValue;
elseif (m_inputValue < k_minValue)
    p_error = 1;
    p_errorMessage = k_valueNameString;
    p_output = k_maxValue;
else
    p_output = m_inputValue;
    p_error = 0;
    p_errorMessage = 0;
end

== stateflow chart Assignment_2_PacemakerProjRA/Data Processing/Chart ==
  settings: executeAtInitialization=1
  state WRITE_STATE
    % This state is triggered when 2nd byte == 20
    entry:
    % Edit all values based on input from UART0
    p_mode = rxdata(3);
    p_activityThreshold = rxdata(4);
    p_arp = typecast(rxdata(5:6), 'uint16');
    p_atrialAmplitude = typecast(rxdata(7:8), 'uint16');
    p_atrialPulseWidth = typecast(rxdata(9:10), 'uint16');
    p_hysteresis = rxdata(11);
    p_hysteresisLimit = rxdata(12);
    p_maximumSensorRate = rxdata(13);
    p_lowrateLimit = rxdata(14);
    p_reactionTime = rxdata(15);
    p_recoveryTime = rxdata(16);
    p_responseFactor = rxdata(17);
    p_upperrateLimit = rxdata(18);
    p_ventricularAmplitude = typecast(rxdata(19:20), 'uint16');
    p_ventricularPulseWidth = typecast(rxdata(21:22), 'uint16');
    p_vrp = typecast(rxdata(23:24), 'uint16');
    % Light flashes to show what's happening
    p_blue = 1;
  state DEFAULT
    entry:
    % These default specifications are taken from
    % Appendix A in the PACEMAKER Document
    p_mode = 1;
    p_lowrateLimit = 60;
    p_upperrateLimit = 120;
    p_maximumSensorRate = 120;
    p_atrialAmplitude = uint16(3500);
    p_ventricularAmplitude = uint16(3500);
    p_atrialPulseWidth = uint16(400);
    p_ventricularPulseWidth = uint16(400);
    p_arp = uint16(320);
    p_vrp = uint16(250);
    p_activityThreshold = 3;
    p_reactionTime = 30;
    p_responseFactor = 8;
    p_recoveryTime = 5;
    p_hysteresis = 0;
    p_hysteresisLimit = 30;
  state ECHO_STATE
    % This state is triggered when
    % 2nd byte == 16
    entry:
    % Trigger function to echo
    % values to DCM
    echo_params_alt();
    p_red = 1;
  state BUFFER
    % Waiting for UART
    entry:
    p_red = 0;
    p_blue = 0;
    p_green = 0;
  state EGRAM_STATE
    % This state is triggered when
    % 2nd byte == 22
    entry:
    % Trigger function to send
    % egram data to DCM
    echo_params_alt();
    p_green = 1;
  (default) -> DEFAULT
  WRITE_STATE -> BUFFER
  (junction 55) -> WRITE_STATE [order 2] : [rxdata(2) == hex2dec('20')]
  DEFAULT -> BUFFER
  BUFFER -> (junction 68) : [status == 0]
  (junction 68) -> (junction 55) : [rxdata(1) == hex2dec('16')]
  (junction 55) -> ECHO_STATE [order 1] : [rxdata(2) == hex2dec('16')]
  (junction 55) -> EGRAM_STATE [order 3] : [rxdata(2) == hex2dec('22')]
  EGRAM_STATE -> BUFFER
  ECHO_STATE -> BUFFER
  data: p_activityThreshold output uint8; p_arp output uint16; p_atrialAmplitude output uint16; rxdata input uint8; status input uint8; p_atrialPulseWidth output uint16; p_hysteresis output uint8; p_hysteresisLimit output uint8; p_maximumSensorRate output uint8; p_lowrateLimit output uint8; p_mode output uint8; p_reactionTime output uint8; p_recoveryTime output uint8; p_responseFactor output uint8; p_upperrateLimit output uint8; p_ventricularAmplitude output uint16; p_ventricularPulseWidth output uint16; p_vrp output uint16; p_red output; p_green output; p_blue output

== matlab function Assignment_2_PacemakerProjRA/MATLAB Function1 ==
  data: u input; y output
function y = fcn(u)

y = sum(u) / 3;

== stateflow chart Assignment_2_PacemakerProjRA/Write Mode ==
  state WRITE_MODE
    entry:
    writeModeOutput = 1;
  state INITIAL
    entry:
    writeModeOutput = 0;
  state BUFFER
    entry:
    writeModeOutput = 0;
  (default) -> INITIAL
  INITIAL -> WRITE_MODE : [writeModeInput > 0]
  BUFFER -> INITIAL : [writeModeInput == 0]
  WRITE_MODE -> BUFFER : after(100, msec)
  data: writeModeOutput output; writeModeInput input

== stateflow chart Assignment_2_PacemakerProjRA/Float Variable6/Chart ==
  state INITIAL
    entry:
    % Set default value in initial
    p_outputValue = k_defaultValue;
  state VALUE_CHANGED
    entry:
    % Change output
    p_outputValue = m_inputValue
  state BUFFER
  (default) -> INITIAL
  BUFFER -> VALUE_CHANGED : [m_valueChange > 0]
  VALUE_CHANGED -> BUFFER : after(1000,msec)
  INITIAL -> BUFFER
  data: k_defaultValue input single; m_inputValue input single; p_outputValue output single; m_valueChange input boolean

== stateflow chart Assignment_2_PacemakerProjRA/AOO/VOO State Diagram ==
  state NO_PACE
    entry:
    s_paceStart = true;
  state PACE
    entry:
    s_paceStart = false;
  (default) -> NO_PACE
  PACE -> NO_PACE : after(p_lowrateInterval, msec)
  NO_PACE -> PACE : after(1, msec)
  data: p_lowrateInterval input; s_paceStart output

== matlab function Assignment_2_PacemakerProjRA/Decode p_pacingMode ==
  data: p_pacingMode input; s_offState output; s_AOOState output; s_VOOState output; s_AAIState output; s_VVIState output; s_AOORState output; s_VOORState output; s_AAIRState output; s_VVIRState output
function [s_offState,s_AOOState, s_VOOState, s_AAIState, s_VVIState, s_AOORState, s_VOORState, s_AAIRState, s_VVIRState] = decodeInputInteger(p_pacingMode)

stateList = zeros(1,9);

stateList(p_pacingMode + 1) = 1;

s_offState = stateList(1);
s_AOOState = stateList(2);
s_VOOState = stateList(3);
s_AAIState = stateList(4);
s_VVIState = stateList(5);
s_AOORState = stateList(6);
s_VOORState = stateList(7);
s_AAIRState = stateList(8);
s_VVIRState = stateList(9);

== stateflow chart Assignment_2_PacemakerProjRA/VVI/AAI State Diagram ==
  state INITIAL_STATE
  state SENSED
  note: Hysteresis
  state HYSTERESIS_STATE
  state PACED
    entry:
    s_paceStart = 1;
    on after(1, msec):
    s_paceStart = 0;
  state REGULAR_STATE
  note: No Hysteresis
  (junction 47) -> SENSED
  REGULAR_STATE -> (junction 47) [order 1] : [m_ventSense]
  HYSTERESIS_STATE -> (junction 47) [order 1] : [m_ventSense]
  (default) -> INITIAL_STATE
  INITIAL_STATE -> PACED
  SENSED -> (junction 59) : after(p_vrp, msec)
  (junction 59) -> HYSTERESIS_STATE [order 1] : [p_hysteresis == 1]
  HYSTERESIS_STATE -> (junction 53) [order 2] : after(p_hysteresisLimit, msec)
  REGULAR_STATE -> (junction 53) [order 2] : after(p_lowrateInterval - p_vrp, msec)
  (junction 53) -> PACED
  (junction 59) -> REGULAR_STATE [order 2]
  PACED -> REGULAR_STATE : after(p_vrp, msec)
  data: p_lowrateInterval input uint16; p_vrp input; s_paceStart output; m_ventSense input; p_hysteresis input; p_hysteresisLimit input
